simulink model "QPSK_cx_noise_m70"  (Simulink 7.0)
settings: Solver=VariableStepDiscrete  StartTime=0.0  StopTime=sim_t  RelTol=1e-3
undefined symbols (not defined in the file or in its folder): get, STqn
libraries: commsink2 x3, commdigbbndpm3 x2, commchan3 x1, commrandsrc2 x1
settings Model: Creator=usuario  LastModifiedBy=cocheca
settings DebuggingCC: SaveWithParameterizedLinksMsg=none  SignalResolutionControl=TryResolveAllWithWarning  MultiTaskDSMMsg=warning  MultiTaskCondExecSysMsg=none
settings RTWCC: IncludeERTFirstTime=on
settings GRTTargetCC: TargetFcnLib=ansi_tfl_tmw.mat

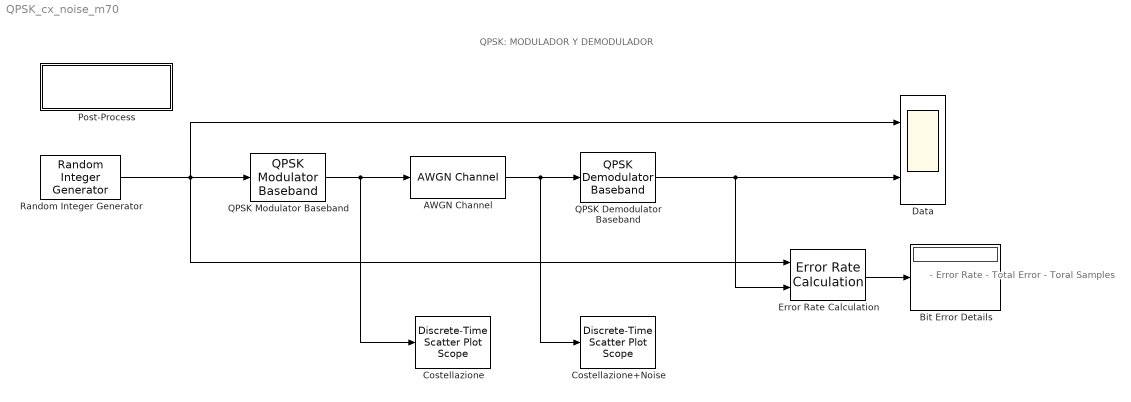
== system QPSK_cx_noise_m70 ==
  note: QPSK: MODULADOR Y DEMODULADOR
  note: - Error Rate
      | - Total Error
      | - Toral Samples
  AWGN Channel : commchan3/AWGN Channel  SystemSampleTime=-1  seed=67  noiseMode="Signal to noise ratio  (SNR)"  EbNodB=20  EsNodB=10  SNRdB=SNRqn  bitsPerSym=1  Ps=1  Tsym=1  variance=1
  Bit Error Details : Display
  Costellazione : commsink2/Discrete-Time Scatter Plot Scope  Tag=ScatterPlot  SystemSampleTime=-1  sampPerSymb=1  offsetEye=0  numTraces=40  numNewFrames=10  LineMarkers=x  LineColors=k  fading=on  render=on  AxisGrid=on  xMin=-3.3  xMax=3.315  yMin=-3.3  yMax=3.315  inphaseLabel=In-phase Amplitude  quadratureLabel=Quadrature Amplitude  openScopeAtSimStart=on  FrameNumber=off  FigPos=get(0,'defaultfigureposition');  figTitle=Scatter Plot  numLinesMax=8  block_type_=scatter
  Costellazione+Noise : commsink2/Discrete-Time Scatter Plot Scope  Tag=ScatterPlot  SystemSampleTime=-1  sampPerSymb=1  offsetEye=0  numTraces=40  numNewFrames=10  LineMarkers=x  LineColors=k  fading=on  render=on  AxisGrid=on  xMin=-3.3  xMax=3.315  yMin=-3.3  yMax=3.315  inphaseLabel=In-phase Amplitude  quadratureLabel=Quadrature Amplitude  openScopeAtSimStart=on  FrameNumber=off  FigPos=get(0,'defaultfigureposition');  figTitle=Scatter Plot  numLinesMax=8  block_type_=scatter
  Data : Scope  NumInputPorts=2
      settings: YMin=-0.5~-0.5  YMax=3.5~3.5
  Error Rate Calculation : commsink2/Error Rate Calculation  N=0  st_delay=0  cp_mode=Entire frame  subframe=[]  PMode=Port  WsName=ErrorVec  RsMode2=off  stop=off  numErr=100  maxBits=1e6
  Post-Process : Subsystem  mask{sim_t=1000, STqn=5, SNRqn=0}
      mask prompts: sim_t "Sim Time [100]"; STqn "Source Sample Time"; SNRqn "SNR"
      mask init:
      | %sim_t = 100; %simulation time
      | %BSTf = 5; % source sample time
      | PZfn = .4; % probability of zero
      | 
      | %STf = 1/100; % sample time
      | %A1f = 1; % amplitude sine 1 - mod.
      | %A2f = 1; % amplitude sine 2 - mod.
      | %F1f = 2*pi*8; % Freg Sine 1
      | %F2f = 2*pi*12; % Freg Sine 2
      | 
      | 
      | % Sample Time Source Configure
      | switch STqn
      |     case 1
      |         STqn = 1;
      |     case 2
      |         STqn = 5;
      |     case 3
      |         STqn = 10;      
      | end
      | 
      | % switch SNRqn
      | %     case 1
      | %         SNRqn = -10;
      | %     case 2
      | %         SNRqn = -5;
      | %     case 3
      | %         SNRqn = 0;
      | %     case 4
      | %         SNRqn = 5;
      | %     case 5
      | %         SNRqn = 10;        
      | %     case 6
      | %         SNRqn = 20;        
      | % end
      | 
      | switch sim_t
      |     case 1
      |         sim_t = 50;
      |     case 2
      |         sim_t = 100;
      |     case 3
      |         sim_t = 250;
      |     case 4
      |         sim_t = 500;
      |     case 5
      |         sim_t = 1000;        
      | end
      | 
      | assignin('base','sim_t', sim_t );
      | assignin('base','STqn', STqn );
      | assignin('base','SNRqn', SNRqn );
      mask StyleString: popup(50|100|250|500|1000),popup(1|5|10),edit
      mask Display: disp('Sim Parameters')
  QPSK Demodulator Baseband : commdigbbndpm3/QPSK Demodulator Baseband  DialogController=commDDGCreate  DialogControllerArgs=DataTag0  Ph=pi/4  Dec=Gray  OutType=Integer  DecType=Hard decision  VarSource=Dialog  Variance=1  outDtype1=Inherit via internal rule  outDtype2=Inherit via internal rule  derotateFactorWordLen=16
  QPSK Modulator Baseband : commdigbbndpm3/QPSK Modulator Baseband  DialogController=commDDGCreate  DialogControllerArgs=DataTag1  SystemSampleTime=-1  InType=Integer  Enc=Gray  Ph=pi/4  outDtype=double  outWordLen=16  outUDDataType=sfix(16)  outFracLenMode=Best precision  outFracLen=15
  Random Integer Generator : commrandsrc2/Random Integer Generator  SystemSampleTime=-1  mul=4  seed=37  Ts=STqn  frameBased=off  sampPerFrame=1  orient=off  outDataType=double
  wires:
  Random Integer Generator/1 -> Error Rate Calculation/1, QPSK Modulator Baseband/1, Data/1
  QPSK Modulator Baseband/1 -> AWGN Channel/1, Costellazione/1
  AWGN Channel/1 -> QPSK Demodulator Baseband/1, Costellazione+Noise/1
  QPSK Demodulator Baseband/1 -> Error Rate Calculation/2, Data/2
  Error Rate Calculation/1 -> Bit Error Details/1

== system QPSK_cx_noise_m70/Post-Process ==
